simulink model "AcO_Ctrl_Geometric_headless_R2016a"  (R2016a)
settings: Solver=FixedStepDiscrete  StartTime=0.0  StopTime=simulation_duration  FixedStep=Ts  RelTol=1e-3
values from neighbouring files (symbols this model uses):
  M1_BeMo_d = zeros(7,M1_n_mode)    [AcO_Ctrl_headless_cfg.m]    (also in agws_cfg.m = 1e-6*bsxfun(@times,randn(7,M1_n_mode),scale); agws_fastTT_cfg.m = 1e-6*bsxfun(@times,randn(7,M1_n_mode),scale))
  M1_RiBo_d = zeros(7,6)    [AcO_Ctrl_headless_cfg.m]    (also in agws_cfg.m = [M1_Txyz0 M1_Rxyz0]; agws_fastTT_cfg.m = [M1_Txyz0 M1_Rxyz0])
  M2_RiBo_d = zeros(7,6)    [AcO_Ctrl_headless_cfg.m]    (also in agws_cfg.m = [M2_Txyz0 M2_Rxyz0]; agws_fastTT_cfg.m = [M2_Txyz0 M2_Rxyz0])
  Ts = 1/fs    (= 0.002)    [AcO_Ctrl_headless_cfg.m]    (also in agws_fastTT_cfg.m = 0.005)
undefined symbols (not defined in the file or in its folder): Az_C, CG2Hp, CG2Hp_S7, El_C, Fsmm, GIR_C, Hp2CG_f, Hp2CG_f_S7, HPdtf, HpK, KM2, M2_actdyn, M2_CG2Hp, M_LOS, MIMO_C, PTT2act, PTT2act_even, Q, sysd, TT2act, TT2act_even
undefined symbols (not defined in the file): on_axis_src_outputs
libraries: CEO x2
(part 1 of 6)
settings Model: Creator=rconan  LastModifiedBy=rconan
settings DataIOCC: LimitDataPoints=on  SaveFormat=Array
settings OptimizationCC: EfficientMapNaN2IntZero=off
settings HardwareCC: ProdBitPerPointer=32  ProdLargestAtomicFloat=None  ProdIntDivRoundTo=Undefined  ProdEndianess=Unspecified  ProdWordSize=32  ProdHWDeviceType=32-bit Generic  TargetBitPerLong=64  TargetBitPerPointer=64  TargetLongLongMode=on  TargetIntDivRoundTo=Zero  TargetEndianess=LittleEndian  TargetWordSize=64  TargetHWDeviceType=MATLAB Host  ProdEqTarget=off
settings ModelReferenceCC: PropagateSignalLabelsOutOfModel=off
settings CodeAppCC: MaxIdLength=128
settings GRTTargetCC: GeneratePreprocessorConditionals=Use local settings  CombineOutputUpdateFcns=off  GRTInterface=on

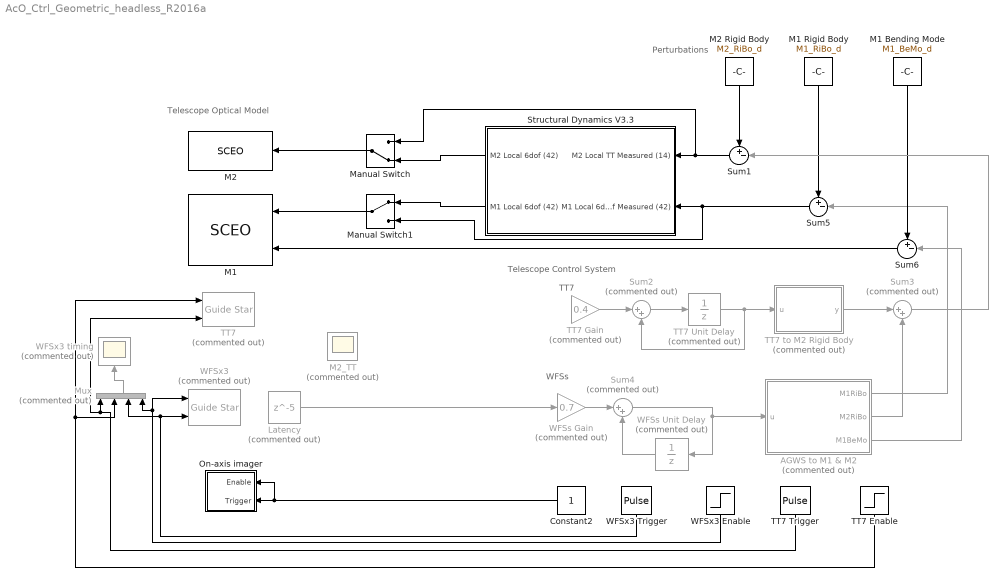
== system AcO_Ctrl_Geometric_headless_R2016a ==
  note: TT7
  note: WFSs
  note: Perturbations
  note: Telescope Control System
  note: Telescope Optical Model
  AGWS to M1 & M2 : MATLAB Function  Commented=on  TreatAsAtomicUnit=on
  Constant2 : Constant  SampleTime=Inf
  Latency : Delay  Commented=on  DelayLength=5
  M1 : M-S-Function  AncestorBlock=CEO/M1 or M2  FunctionName=SCEO  mask(GMTMirror){mirror=M1, TxyzRxyz=on, mode_coefs=on, n_mode=42, sampleTime=[-1,0]}
      mask prompts: TxyzRxyz "Txyz and Rxyz rigid body"; mode_coefs "Mirror mode coefficients"; sampleTime "Sample Time"
      mask help: The GMT M1 or M2 model
      mask init:
      | class_id = 'GMT';
      | msg_box = ceo.dealer(class_id,get_param(gcb,'Name'));
      | set(gcbh,'UserData',msg_box)
      | mask = Simulink.Mask.get(gcb);
      | n_in = 2;
      | msg_box.sampleTime = sampleTime;
      | 
      | gmt_mirror = get_param(gcb,'mirror');
      | 
      | %% START
      | if strcmp(gmt_mirror,'M1')
      |     mirror_args = struct(...
      |         'mirror_modes','bending modes',...
      |         'N_MODE',n_mode);
      |     dims_in = {[7,6],[7,n_mode]};
      | else
      |     mirror_args = struct(...
      |         'mirror_modes','Karhunen-Loeve',...
      |         'N_MODE',n_mode);
      |     dims_in = {[7,6],[7,n_mode]};
      | end
      | start_args = struct('mirror',gmt_mirror,'mirror_args',mirror_args);
      | msg_box.start.args = start_args;
      |          
      | %% UPDATE
      | n_in = 0;
      | inputs_args = struct();
      | update_args = struct('mirror',gmt_mirror,'inputs_args',inputs_args);
      | if TxyzRxyz
      |     n_in = n_in + 1;
      |     dims_in{n_in} = [7,6];
      |     update_args.inputs_args.('TxyzRxyz') = [];
      | end
      | if mode_coefs
      |     n_in = n_in + 1;
      |     dims_in{n_in} = [7,n_mode];
      |     update_args.inputs_args.('mode_coefs') = [];
      | end
      | msg_box.n_in = n_in;
      | msg_box.n_in_ceo = n_in;
      | msg_box.dims_in = dims_in;
      | msg_box.update.args = update_args;
      | 
      | %% OUTPUTS
      | msg_box.n_out = 0;
      | msg_box.dims_out = [];
      mask Help: web(fullfile(fileparts(which('SCEO')),'masks',[get_param(gcb,'MaskType'),'.html']))
      mask TypeOptions mirror: M1 | M2
      mask DialogControl DescGroupVar Prompt: GMT M1 or M2 segmented mirror
      mask DialogControl DescTextVar Prompt: Select to command either M1 or M2 degrees of freedom
      mask DialogControl mirror_commnand Prompt: Mirror commands
      mask Display: fprintf('GMT\nMirror')
  M1 Bending Mode : Constant  Value=M1_BeMo_d
  M1 Rigid Body : Constant  Value=M1_RiBo_d
  M2 : M-S-Function  AncestorBlock=CEO/M1 or M2  FunctionName=SCEO  mask(GMTMirror){mirror=M2, TxyzRxyz=on, mode_coefs=off, n_mode=66, sampleTime=[-1,0]}
      mask prompts: TxyzRxyz "Txyz and Rxyz rigid body"; mode_coefs "Mirror mode coefficients"; sampleTime "Sample Time"
      mask help: The GMT M1 or M2 model
      mask init: same as AcO_Ctrl_Geometric_headless_R2016a/M1
      mask Help: web(fullfile(fileparts(which('SCEO')),'masks',[get_param(gcb,'MaskType'),'.html']))
      mask TypeOptions mirror: M1 | M2
      mask DialogControl DescGroupVar Prompt: GMT M1 or M2 segmented mirror
      mask DialogControl DescTextVar Prompt: Select to command either M1 or M2 degrees of freedom
      mask DialogControl mirror_commnand Prompt: Mirror commands
      mask Display: fprintf('GMT\nMirror')
  M2 Rigid Body : Constant  Value=M2_RiBo_d
  M2_TT : Scope  Commented=on
  Manual Switch : ManualSwitch  CurrentSetting=0
  Manual Switch1 : ManualSwitch
  Mux : Mux  Commented=on
  On-axis imager : Subsystem
  Structural Dynamics V3.3 : Subsystem  Variant=on
  Sum1 : Sum  Inputs=+-|
  Sum2 : Sum  Commented=on  Inputs=|++
  Sum3 : Sum  Commented=on  Inputs=|++
  Sum4 : Sum  Commented=on  Inputs=|++
  Sum5 : Sum  Inputs=+-|
  Sum6 : Sum  Inputs=+-|
  TT7 : CEO/Guide Star  Commented=on  source_prm='JSON/AcO_Ctrl/AcO_TT7_GUIDE_STAR.ubj'  sensor=GeometricTT7  sensor_prm='JSON/AcO_Ctrl/AcO_TT7.ubj'  sensor_calib=tt7_calib  sensor_out={{'M2_TT',14}}  sampleTime=[Ts,0]
  TT7 Trigger : DiscretePulseGenerator  Period=3  PhaseDelay=1/Ts + 3  SampleTime=Ts
  TT7 Enable : Step  SampleTime=Ts
  TT7 Gain : Gain  Commented=on  Gain=0.4
  TT7 Unit Delay : UnitDelay  Commented=on  SampleTime=-1
  TT7 to M2 Rigid Body : MATLAB Function  Commented=on  TreatAsAtomicUnit=on
  WFSs Unit Delay : UnitDelay  Commented=on  SampleTime=-1
  WFSs Gain : Gain  Commented=on  Gain=0.7
  WFSx3 : CEO/Guide Star  Commented=on  source_prm='JSON/AcO_Ctrl/AcO_WFS_GUIDE_STARS.ubj'  sensor=GeometricShackHartmann  sensor_prm='JSON/AcO_Ctrl/AcO_WFS.ubj'  sensor_calib=gs_calib  sensor_out={{'AGWS_D',gs_calib_size}}  sampleTime=[Ts,0]
  WFSx3 Enable : Step  Time=1.5  SampleTime=Ts
  WFSx3 Trigger : DiscretePulseGenerator  Period=0.5/Ts  PhaseDelay=2/Ts  SampleTime=Ts
  WFSx3 timing : Scope  Commented=on
  wires:
  TT7 Unit Delay/1 -> Sum2/2, TT7 to M2 Rigid Body/1(u)
  Sum2/1 -> TT7 Unit Delay/1
  TT7 Gain/1 -> Sum2/1
  Constant2/1 -> On-axis imager/1(Enable), On-axis imager/2(Trigger)
  Mux/1 -> WFSx3 timing/1
  TT7 Trigger/1 -> TT7/2, Mux/1
  TT7 to M2 Rigid Body/1(y) -> Sum3/1
  AGWS to M1 & M2/2(M2RiBo) -> Sum3/2
  Sum4/1 -> WFSs Unit Delay/1, AGWS to M1 & M2/1(u)
  ? -> Latency/1  "AGWS_D"
  WFSs Gain/1 -> Sum4/1
  AGWS to M1 & M2/1(M1RiBo) -> Sum5/2
  M1 Rigid Body/1 -> Sum5/1
  WFSx3 Enable/1 -> Mux/4, WFSx3/1
  AGWS to M1 & M2/3(M1BeMo) -> Sum6/2
  M1 Bending Mode/1 -> Sum6/1
  WFSx3 Trigger/1 -> Mux/3, WFSx3/2
  ? -> TT7 Gain/1, M2_TT/1  "M2_TT"
  Latency/1 -> WFSs Gain/1
  WFSs Unit Delay/1 -> Sum4/2
  Sum5/1 -> Manual Switch1/2, Structural Dynamics V3.3/2(M1 Local 6dof Measured (42))
  Manual Switch/1 -> M2/1
  Manual Switch1/1 -> M1/1
  Sum1/1 -> Manual Switch/1, Structural Dynamics V3.3/1(M2 Local TT Measured (14))
  M2 Rigid Body/1 -> Sum1/1
  TT7 Enable/1 -> Mux/2, TT7/1
  Structural Dynamics V3.3/1(M2 Local 6dof (42)) -> Manual Switch/2
  Structural Dynamics V3.3/2(M1 Local 6dof (42)) -> Manual Switch1/1
  Sum3/1 -> Sum1/2
  Sum6/1 -> M1/2

== system AcO_Ctrl_Geometric_headless_R2016a/On-axis imager ==
  Enable : Inport  SampleTime=Ts
  Trigger : Inport  Port=2  SampleTime=Ts
  Bus Creator : BusCreator  Inputs=5
  Science Star : M-S-Function  AncestorBlock=CEO/Guide Star  FunctionName=SCEO  mask(OpticalPath){source_prm='JSON/AcO_Ctrl/AcO_ON_AXIS_SRC.ubj', sensor=Imaging, sensor_prm='JSON/AcO_Ctrl/AcO_ON_AXIS_IMGR.ubj', sensor_calib=struct('calibrations',[],'filename',[],'pseudo_inverse',[]), sensor_out=on_axis_src_outputs, sampleTime=[Ts,0]}
      mask prompts: source_prm "Parameters"; sensor "Type"; sensor_prm "Parameters"; sensor_calib "Calibration"; sensor_out "Outputs"; sampleTime "Sample Time"
      mask help: Generate a Guide Star and an optional optical sensor
      mask init:
      | class_id = 'OP';
      | msg_box = ceo.dealer(class_id,get_param(gcb,'Name'));
      | set(gcbh,'UserData',msg_box)
      | mask = Simulink.Mask.get(gcb);
      | n_in = 2;
      | dims_in = [];
      | msg_box.n_in = n_in;
      | msg_box.n_in_ceo = 0;
      | msg_box.dims_in = {1,1};
      | n_out = 0;
      | dims_out = {};
      | msg_box.sampleTime = sampleTime;
      | %% START
      | % Source
      | source_args = ceo.liftprm(source_prm);
      | % Sensor
      | prm = mask.getParameter('sensor');
      | sensor_class = prm.TypeOptions{sensor};
      | sensor_args = ceo.liftprm(sensor_prm);
      | miscellaneous_args = [];
      | calib_src_args = [];
      | start_args = struct('source_args',source_args,...
      |               'sensor_class',sensor_class,...
      |               'sensor_args',sensor_args,...
      |               'calibration_source_args',calib_src_args,...
      |               'miscellaneous_args',miscellaneous_args);
      | msg_box.start.args = start_args;
      | %% UPDATE
      | update_args = struct('inputs',[]);
      | msg_box.update.args = update_args;
      | %% OUTPUTS
      | if isempty(sensor_out)
      |     outputs_args = struct('outputs',{[]});
      | else
      |     outputs_args = struct('outputs',{cellfun(@(x) x(1) , sensor_out)} );
      |     dims_out = cellfun(@(x) x(2) , sensor_out );
      |     n_out = numel(dims_out);
      | end
      | msg_box.n_out = n_out;
      | msg_box.dims_out = dims_out;
      | msg_box.outputs.args = outputs_args;
      | %% INITIALIZECONDITIONS
      | init_args = ceo.liftprm(sensor_calib);
      | msg_box.init.args = init_args;
      | 
      | dump(msg_box)
      mask Help: web(fullfile(fileparts(which('SCEO')),'masks',[get_param(gcb,'MaskType'),'.html']))
      mask TypeOptions sensor: None | Imaging | ShackHartmann | GeometricShackHartmann | GeometricTT7
      mask DialogControl DescGroupVar Prompt: Optical Path
      mask DialogControl DescTextVar Prompt: An optical path through the telescope consists in a star and a sensor. Ray tracing is performed from the star to the exist pupil of the GMT. From the exist pupil, the wavefront of the star is Fourier propagated to the detector plane of the sensor.
      mask DialogControl Container14 Prompt: Source
      mask DialogControl Container18 Prompt: Sensor
      mask Display: fprintf('Optical\nPath')
  To File : ToFile  Filename=metrics_MDL353_CASE2_PATCH4.mat  MatrixName=metrics  SaveFormat=Timeseries
  wires:
  Science Star/3 -> Bus Creator/3  "segment_piston"
  Science Star/5 -> Bus Creator/5  "segment_tiptilt"
  Science Star/2 -> Bus Creator/2  "segment_wfe_rms"
  Science Star/1 -> Bus Creator/1  "wfe_rms"
  Enable/1 -> Science Star/1
  Trigger/1 -> Science Star/2
  Science Star/4 -> Bus Creator/4  "tiptilt"
  Bus Creator/1 -> To File/1

== system AcO_Ctrl_Geometric_headless_R2016a/Structural Dynamics V3.3 ==
  M2 Local TT Measured (14) : Inport
  M1 Local 6dof Measured (42) : Inport  Port=2
  Structural Dynamics V3.1 : Subsystem  VariantControl=STATE_SPACE_MDL==310
  Structural Dynamics V3.3 : Subsystem  VariantControl=STATE_SPACE_MDL==330
  Structural Dynamics V3.3a : Subsystem  VariantControl=STATE_SPACE_MDL==331
  Structural Dynamics V3.5.2 : Subsystem  VariantControl=STATE_SPACE_MDL==352
  Structural Dynamics V3.5.3 : Subsystem  VariantControl=STATE_SPACE_MDL==353
  M2 Local 6dof (42) : Outport
  M1 Local 6dof (42) : Outport  Port=2

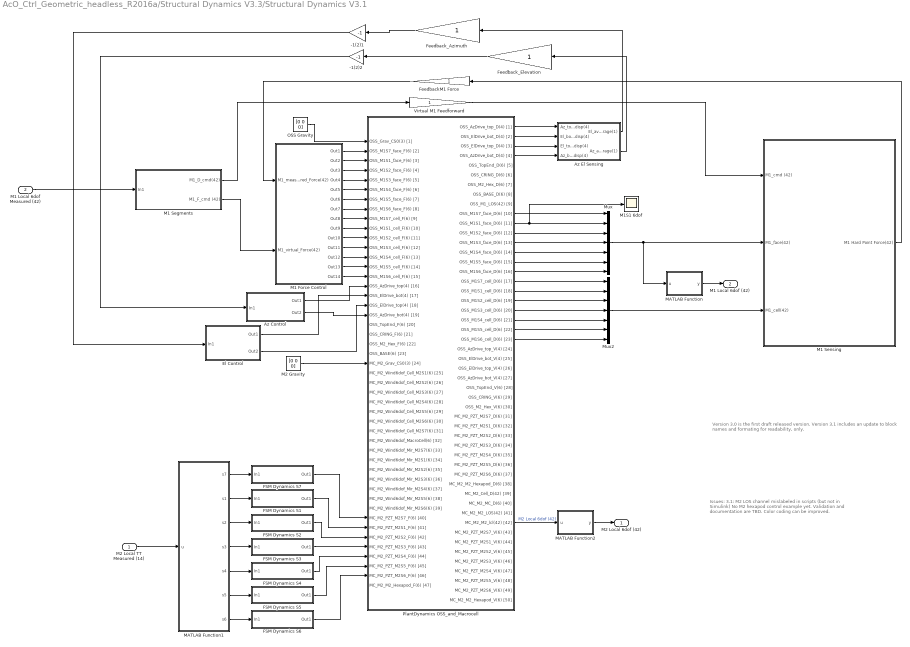
== system AcO_Ctrl_Geometric_headless_R2016a/Structural Dynamics V3.3/Structural Dynamics V3.1 ==
  note: Version 3.0 is  the first draft released version.
      | Version 3.1 includes an update to block names and formating for readability, only.
  note: Issues:
      | 3.1:
      | M2 LOS channel mislabeled in scripts (but not in Simulink)
      | No M2 hexapod control example yet.
      | Validation and documentation are TBD.
      | Color coding can be improved.
  M2 Local TT Measured (14) : Inport
  M1 Local 6dof Measured (42) : Inport  Port=2
  -1(2)1 : Gain  Gain=-1
  -1(2)2 : Gain  Gain=-1
  Az Control : Subsystem
  Az El Sensing : Subsystem
  El Control : Subsystem
  FSM Dynamics S1 : Subsystem
  FSM Dynamics S2 : Subsystem
  FSM Dynamics S3 : Subsystem
  FSM Dynamics S4 : Subsystem
  FSM Dynamics S5 : Subsystem
  FSM Dynamics S6 : Subsystem
  FSM Dynamics S7 : Subsystem
  FeedbackM1 Force : Gain
  Feedback_Azimuth : Gain
  Feedback_Elevation : Gain
  M1 Force Control : Subsystem
  M1 Segments : Subsystem
  M1 Sensing : Subsystem
  M1S1 6dof : Scope
  M2 Gravity : Constant  Value=[0 0 0]
  MATLAB Function : MATLAB Function  TreatAsAtomicUnit=on
  MATLAB Function1 : MATLAB Function  TreatAsAtomicUnit=on
  MATLAB Function2 : MATLAB Function  TreatAsAtomicUnit=on
  Mux : Mux  Inputs=6*ones(7,1)
  Mux2 : Mux  Inputs=6*ones(7,1)
  OSS Gravity : Constant  Value=[0 0 0]
  PlantDynamics OSS_and_Macrocell : Subsystem
  Virtual M1 Feedforward : Gain
  M2 Local 6dof (42) : Outport
  M1 Local 6dof (42) : Outport  Port=2
  wires:
  M2 Local TT Measured (14)/1 -> MATLAB Function1/1(u)
  FSM Dynamics S7/1(Out1) -> PlantDynamics OSS_and_Macrocell/40(MC_M2_PZT_M2S7_F(6) [40])
  MATLAB Function2/1(y) -> M2 Local 6dof (42)/1
  MATLAB Function/1(y) -> M1 Local 6dof (42)/1
  M1 Local 6dof Measured (42)/1 -> M1 Segments/1(In1)
  MATLAB Function1/1(s7) -> FSM Dynamics S7/1(In1)
  MATLAB Function1/2(s1) -> FSM Dynamics S1/1(In1)
  MATLAB Function1/3(s2) -> FSM Dynamics S2/1(In1)
  MATLAB Function1/4(s3) -> FSM Dynamics S3/1(In1)
  MATLAB Function1/5(s4) -> FSM Dynamics S4/1(In1)
  MATLAB Function1/6(s5) -> FSM Dynamics S5/1(In1)
  MATLAB Function1/7(s6) -> FSM Dynamics S6/1(In1)
  Virtual M1 Feedforward/1 -> M1 Sensing/1(M1_cmd (42))
  Az El Sensing/2(Az_average(1)) -> Feedback_Elevation/1
  Az El Sensing/1(El_average(1)) -> Feedback_Azimuth/1
  PlantDynamics OSS_and_Macrocell/4(OSS_AzDrive_bot_D(4) [4]) -> Az El Sensing/4(Az_bot_disp(4))
  PlantDynamics OSS_and_Macrocell/3(OSS_ElDrive_top_D(4) [3]) -> Az El Sensing/3(El_top_disp(4))
  PlantDynamics OSS_and_Macrocell/2(OSS_ElDrive_bot_D(4) [2]) -> Az El Sensing/2(El_bottom_disp(4))
  PlantDynamics OSS_and_Macrocell/1(OSS_AzDrive_top_D(4) [1]) -> Az El Sensing/1(Az_top_disp(4))
  M1 Segments/2(M1_F_cmd (42)) -> M1 Force Control/2(M1_virtual_Force(42))
  M1 Segments/1(M1_D_cmd(42)) -> Virtual M1 Feedforward/1
  M1 Force Control/14(Out14) -> PlantDynamics OSS_and_Macrocell/15(OSS_M1S6_cell_F(6) [15])
  M1 Force Control/13(Out13) -> PlantDynamics OSS_and_Macrocell/14(OSS_M1S5_cell_F(6) [14])
  M1 Force Control/12(Out12) -> PlantDynamics OSS_and_Macrocell/13(OSS_M1S4_cell_F(6) [13])
  M1 Force Control/11(Out11) -> PlantDynamics OSS_and_Macrocell/12(OSS_M1S3_cell_F(6) [12])
  M1 Force Control/10(Out10) -> PlantDynamics OSS_and_Macrocell/11(OSS_M1S2_cell_F(6) [11])
  M1 Force Control/9(Out9) -> PlantDynamics OSS_and_Macrocell/10(OSS_M1S1_cell_F(6) [10])
  M1 Force Control/8(Out8) -> PlantDynamics OSS_and_Macrocell/9(OSS_M1S7_cell_F(6) [9])
  M1 Force Control/7(Out7) -> PlantDynamics OSS_and_Macrocell/8(OSS_M1S6_face_F(6) [8])
  M1 Force Control/6(Out6) -> PlantDynamics OSS_and_Macrocell/7(OSS_M1S5_face_F(6) [7])
  M1 Force Control/5(Out5) -> PlantDynamics OSS_and_Macrocell/6(OSS_M1S4_face_F(6) [6])
  M1 Force Control/4(Out4) -> PlantDynamics OSS_and_Macrocell/5(OSS_M1S3_face_F(6) [5])
  M1 Force Control/3(Out3) -> PlantDynamics OSS_and_Macrocell/4(OSS_M1S2_face_F(6) [4])
  M1 Force Control/2(Out2) -> PlantDynamics OSS_and_Macrocell/3(OSS_M1S1_face_F(6) [3])
  M1 Force Control/1(Out1) -> PlantDynamics OSS_and_Macrocell/2(OSS_M1S7_face_F(6) [2])
  FeedbackM1 Force/1 -> M1 Force Control/1(M1_measured_Force(42))
  El Control/2(Out2) -> PlantDynamics OSS_and_Macrocell/18(OSS_ElDrive_top(4) [18])
  El Control/1(Out1) -> PlantDynamics OSS_and_Macrocell/17(OSS_ElDrive_bot(4) [17])
  -1(2)1/1 -> El Control/1(In1)
  Az Control/2(Out2) -> PlantDynamics OSS_and_Macrocell/19(OSS_AzDrive_bot(4) [19])
  Az Control/1(Out1) -> PlantDynamics OSS_and_Macrocell/16(OSS_AzDrive_top(4) [16])
  -1(2)2/1 -> Az Control/1(In1)
  M1 Sensing/1(M1 Hard Point Force(42)) -> FeedbackM1 Force/1
  Mux2/1 -> M1 Sensing/3(M1_cell(42))
  PlantDynamics OSS_and_Macrocell/23(OSS_M1S6_cell_D(6) [23]) -> Mux2/7
  PlantDynamics OSS_and_Macrocell/22(OSS_M1S5_cell_D(6) [22]) -> Mux2/6
  PlantDynamics OSS_and_Macrocell/21(OSS_M1S4_cell_D(6) [21]) -> Mux2/5
  PlantDynamics OSS_and_Macrocell/20(OSS_M1S3_cell_D(6) [20]) -> Mux2/4
  PlantDynamics OSS_and_Macrocell/19(OSS_M1S2_cell_D(6) [19]) -> Mux2/3
  PlantDynamics OSS_and_Macrocell/18(OSS_M1S1_cell_D(6) [18]) -> Mux2/2
  PlantDynamics OSS_and_Macrocell/17(OSS_M1S7_cell_D(6) [17]) -> Mux2/1
  PlantDynamics OSS_and_Macrocell/15(OSS_M1S5_face_D(6) [15]) -> Mux/6
  PlantDynamics OSS_and_Macrocell/12(OSS_M1S2_face_D(6) [12]) -> Mux/3
  PlantDynamics OSS_and_Macrocell/11(OSS_M1S1_face_D(6) [11]) -> Mux/2, M1S1 6dof/1
  PlantDynamics OSS_and_Macrocell/14(OSS_M1S4_face_D(6) [14]) -> Mux/5
  PlantDynamics OSS_and_Macrocell/16(OSS_M1S6_face_D(6) [16]) -> Mux/7
  PlantDynamics OSS_and_Macrocell/13(OSS_M1S3_face_D(6) [13]) -> Mux/4
  PlantDynamics OSS_and_Macrocell/10(OSS_M1S7_face_D(6) [10]) -> Mux/1
  FSM Dynamics S6/1(Out1) -> PlantDynamics OSS_and_Macrocell/46(MC_M2_PZT_M2S6_F(6) [46])
  FSM Dynamics S5/1(Out1) -> PlantDynamics OSS_and_Macrocell/45(MC_M2_PZT_M2S5_F(6) [45])
  FSM Dynamics S4/1(Out1) -> PlantDynamics OSS_and_Macrocell/44(MC_M2_PZT_M2S4_F(6) [44])
  FSM Dynamics S3/1(Out1) -> PlantDynamics OSS_and_Macrocell/43(MC_M2_PZT_M2S3_F(6) [43])
  FSM Dynamics S2/1(Out1) -> PlantDynamics OSS_and_Macrocell/42(MC_M2_PZT_M2S2_F(6) [42])
  FSM Dynamics S1/1(Out1) -> PlantDynamics OSS_and_Macrocell/41(MC_M2_PZT_M2S1_F(6) [41])
  PlantDynamics OSS_and_Macrocell/42(MC_M2_M2_lcl(42) [42]) -> MATLAB Function2/1(u)  "M2 Local 6dof (42)"
  Mux/1 -> M1 Sensing/2(M1_face(42)), MATLAB Function/1(u)
  Feedback_Elevation/1 -> -1(2)2/1
  Feedback_Azimuth/1 -> -1(2)1/1
  M2 Gravity/1 -> PlantDynamics OSS_and_Macrocell/24(MC_M2_Grav_CS0(3) [24])
  OSS Gravity/1 -> PlantDynamics OSS_and_Macrocell/1(OSS_Grav_CS0(3) [1])

== system AcO_Ctrl_Geometric_headless_R2016a/Structural Dynamics V3.3/Structural Dynamics V3.3 ==
  M2 Local TT Measured (14) : Inport
  M1 Local 6dof Measured (42) : Inport  Port=2
  Loads : Subsystem
  MATLAB Function : MATLAB Function  TreatAsAtomicUnit=on
  MATLAB Function1 : MATLAB Function  TreatAsAtomicUnit=on
  MATLAB Function2 : MATLAB Function  TreatAsAtomicUnit=on
  MC_CEO : Constant  Value=[0;0;0;0;0;0]
  Structural Dynamics Plus CL Az El M1 force : Subsystem
  TT2PTT : MATLAB Function  TreatAsAtomicUnit=on
  M2 Local 6dof (42) : Outport
  M1 Local 6dof (42) : Outport  Port=2
  wires:
  MATLAB Function1/1(y) -> M2 Local 6dof (42)/1
  MATLAB Function/1(y) -> M1 Local 6dof (42)/1
  M2 Local TT Measured (14)/1 -> TT2PTT/1(u)
  Structural Dynamics Plus CL Az El M1 force/1(M1_displacement_lcl(42)) -> MATLAB Function/1(u)
  Structural Dynamics Plus CL Az El M1 force/2(M2 Displacement (segment local) (42)) -> MATLAB Function1/1(u)
  M1 Local 6dof Measured (42)/1 -> MATLAB Function2/1(u)
  MC_CEO/1 -> Structural Dynamics Plus CL Az El M1 force/3(M2 Hexapod Reference M2 Local (6))
  TT2PTT/1(y) -> Structural Dynamics Plus CL Az El M1 force/4(Tip Tilt actuator reference (segment Local) (3))
  Loads/1(Out1) -> Structural Dynamics Plus CL Az El M1 force/1(Loads (111))
  MATLAB Function2/1(y) -> Structural Dynamics Plus CL Az El M1 force/2(M1_reference (42))

== system AcO_Ctrl_Geometric_headless_R2016a/Structural Dynamics V3.3/Structural Dynamics V3.3a ==
  M2 Local TT Measured (14) : Inport
  M1 Local 6dof Measured (42) : Inport  Port=2
  Loads : Subsystem
  MATLAB Function : MATLAB Function  TreatAsAtomicUnit=on
  MATLAB Function1 : MATLAB Function  TreatAsAtomicUnit=on
  MATLAB Function2 : MATLAB Function  TreatAsAtomicUnit=on
  MC_CEO : Constant  Value=[0;0;0;0;0;0]
  Structural Dynamics Plus CL Az El M1 force : Subsystem
  TT2PTT : MATLAB Function  TreatAsAtomicUnit=on
  M2 Local 6dof (42) : Outport
  M1 Local 6dof (42) : Outport  Port=2
  wires:
  MATLAB Function1/1(y) -> M2 Local 6dof (42)/1
  MATLAB Function/1(y) -> M1 Local 6dof (42)/1
  M2 Local TT Measured (14)/1 -> TT2PTT/1(u)
  Structural Dynamics Plus CL Az El M1 force/1(M1_displacement_lcl(42)) -> MATLAB Function/1(u)
  Structural Dynamics Plus CL Az El M1 force/2(M2 Displacement (segment local) (42)) -> MATLAB Function1/1(u)
  M1 Local 6dof Measured (42)/1 -> MATLAB Function2/1(u)
  MC_CEO/1 -> Structural Dynamics Plus CL Az El M1 force/3(M2 Hexapod Reference M2 Local (6))
  TT2PTT/1(y) -> Structural Dynamics Plus CL Az El M1 force/4(Tip Tilt actuator reference (segment Local) (3))
  Loads/1(Out1) -> Structural Dynamics Plus CL Az El M1 force/1(Loads (111))
  MATLAB Function2/1(y) -> Structural Dynamics Plus CL Az El M1 force/2(M1_reference (42))

== system AcO_Ctrl_Geometric_headless_R2016a/Structural Dynamics V3.3/Structural Dynamics V3.5.2 ==
  M2 Local TT Measured (14) : Inport
  M1 Local 6dof Measured (42) : Inport  Port=2
  Loads : Constant  Value=zeros(1,141)
  MATLAB Function : MATLAB Function  TreatAsAtomicUnit=on
  MATLAB Function1 : MATLAB Function  TreatAsAtomicUnit=on
  MATLAB Function2 : MATLAB Function  TreatAsAtomicUnit=on
  MC_CEO : Constant  Value=[0;0;0;0;0;0]
  Manual Switch : ManualSwitch
  Structural Dynamics Plus CL Az El M1 force : Subsystem
  TT2PTT : MATLAB Function  TreatAsAtomicUnit=on
  Terminator : Terminator
  Windloads : Subsystem
  M2 Local 6dof (42) : Outport
  M1 Local 6dof (42) : Outport  Port=2
  wires:
  MATLAB Function1/1(y) -> M2 Local 6dof (42)/1
  MATLAB Function/1(y) -> M1 Local 6dof (42)/1
  M2 Local TT Measured (14)/1 -> TT2PTT/1(u)
  Structural Dynamics Plus CL Az El M1 force/1(M1_displacement_lcl(42)) -> MATLAB Function/1(u)
  Structural Dynamics Plus CL Az El M1 force/2(M2 Displacement (segment local) (42)) -> MATLAB Function1/1(u)
  M1 Local 6dof Measured (42)/1 -> MATLAB Function2/1(u)
  MC_CEO/1 -> Structural Dynamics Plus CL Az El M1 force/3(M2 Hexapod Reference M2 Local (6))
  TT2PTT/1(y) -> Structural Dynamics Plus CL Az El M1 force/4(Tip Tilt actuator reference (segment Local) (3))
  MATLAB Function2/1(y) -> Structural Dynamics Plus CL Az El M1 force/2(M1_reference (42))
  Manual Switch/1 -> Structural Dynamics Plus CL Az El M1 force/1(Loads (141))
  Windloads/1(LoadInputs) -> Manual Switch/1
  Structural Dynamics Plus CL Az El M1 force/3(LOS output (21)) -> Terminator/1
  Loads/1 -> Manual Switch/2

== system AcO_Ctrl_Geometric_headless_R2016a/Structural Dynamics V3.3/Structural Dynamics V3.5.3 ==
  M2 Local TT Measured (14) : Inport
  M1 Local 6dof Measured (42) : Inport  Port=2
  Loads : Constant  Value=zeros(1,141)
  MATLAB Function : MATLAB Function  TreatAsAtomicUnit=on
  MATLAB Function1 : MATLAB Function  TreatAsAtomicUnit=on
  MATLAB Function2 : MATLAB Function  TreatAsAtomicUnit=on
  MC_CEO : Constant  Value=[0;0;0;0;0;0]
  Manual Switch : ManualSwitch
  Structural Dynamics Plus CL Az El M1 force : Subsystem
  TT2PTT : MATLAB Function  TreatAsAtomicUnit=on
  Terminator : Terminator
  Windloads : Subsystem
  M2 Local 6dof (42) : Outport
  M1 Local 6dof (42) : Outport  Port=2
  wires:
  MATLAB Function1/1(y) -> M2 Local 6dof (42)/1
  MATLAB Function/1(y) -> M1 Local 6dof (42)/1
  M2 Local TT Measured (14)/1 -> TT2PTT/1(u)
  Structural Dynamics Plus CL Az El M1 force/1(M1_displacement_lcl(42)) -> MATLAB Function/1(u)
  Structural Dynamics Plus CL Az El M1 force/2(M2 Displacement (segment local) (42)) -> MATLAB Function1/1(u)
  M1 Local 6dof Measured (42)/1 -> MATLAB Function2/1(u)
  MC_CEO/1 -> Structural Dynamics Plus CL Az El M1 force/3(M2 Hexapod Reference M2 Local (6))
  TT2PTT/1(y) -> Structural Dynamics Plus CL Az El M1 force/4(Tip Tilt actuator reference (segment Local) (3))
  MATLAB Function2/1(y) -> Structural Dynamics Plus CL Az El M1 force/2(M1_reference (42))
  Manual Switch/1 -> Structural Dynamics Plus CL Az El M1 force/1(Loads (141))
  Windloads/1(LoadInputs) -> Manual Switch/1
  Structural Dynamics Plus CL Az El M1 force/3(LOS output (21)) -> Terminator/1
  Loads/1 -> Manual Switch/2

== system AcO_Ctrl_Geometric_headless_R2016a/Structural Dynamics V3.3/Structural Dynamics V3.1/Az Control ==
  In1 : Inport
  -1(2) : Gain  Gain=-ones(4,1)  Multiplication=Matrix(K*u)
  Azimuth Controller : DiscreteFilter  Numerator=El_C.num{1}  Denominator=El_C.den{1}  SampleTime=1/Fsmm
  DEMUX1 : Gain  Gain=ones(4,1)  Multiplication=Matrix(K*u)
  Out1 : Outport
  Out2 : Outport  Port=2
  wires:
  -1(2)/1 -> Out2/1
  Azimuth Controller/1 -> DEMUX1/1, -1(2)/1
  DEMUX1/1 -> Out1/1
  In1/1 -> Azimuth Controller/1

== system AcO_Ctrl_Geometric_headless_R2016a/Structural Dynamics V3.3/Structural Dynamics V3.1/Az El Sensing ==
  note: Note: units are m, not radians for these loops!
      | These loops delta the top and bottom displacements in tangential direction, and average the results.
  Az_top_disp(4) : Inport
  El_bottom_disp(4) : Inport  Port=2
  El_top_disp(4) : Inport  Port=3
  Az_bot_disp(4) : Inport  Port=4
  Az : Scope
  El : Scope
  Sum2 : Sum  Inputs=-+|
  Sum3 : Sum  Inputs=-+|
  average : Gain  Gain=ones(1,4)/4  Multiplication=Matrix(K*u)
  average1 : Gain  Gain=ones(1,4)/4  Multiplication=Matrix(K*u)
  El_average(1) : Outport
  Az_average(1) : Outport  Port=2
  wires:
  El_top_disp(4)/1 -> Sum2/2
  El_bottom_disp(4)/1 -> Sum2/1
  Sum2/1 -> average/1
  Sum3/1 -> average1/1
  average1/1 -> Az/1, Az_average(1)/1
  Az_bot_disp(4)/1 -> Sum3/1
  Az_top_disp(4)/1 -> Sum3/2
  average/1 -> El_average(1)/1, El/1

== system AcO_Ctrl_Geometric_headless_R2016a/Structural Dynamics V3.3/Structural Dynamics V3.1/El Control ==
  In1 : Inport
  -1 : Gain  Gain=-ones(4,1)  Multiplication=Matrix(K*u)
  DEMUX : Gain  Gain=ones(4,1)  Multiplication=Matrix(K*u)
  Elevation Controller : DiscreteFilter  Numerator=El_C.num{1}  Denominator=El_C.den{1}  SampleTime=1/Fsmm
  Out1 : Outport
  Out2 : Outport  Port=2
  wires:
  In1/1 -> Elevation Controller/1
  DEMUX/1 -> Out2/1
  -1/1 -> Out1/1
  Elevation Controller/1 -> DEMUX/1, -1/1

== system AcO_Ctrl_Geometric_headless_R2016a/Structural Dynamics V3.3/Structural Dynamics V3.1/FSM Dynamics S1 ==
  In1 : Inport
  M2actuatorDyanmics5 : DiscreteStateSpace  A=M2_actdyn.A  B=M2_actdyn.B  C=M2_actdyn.C  D=M2_actdyn.D  SampleTime=1/Fsmm
  TT_to_act5 : Gain  Gain=TT2act  Multiplication=Matrix(K*u)
  delta1 : Gain  Gain=[eye(3);-eye(3)]  Multiplication=Matrix(K*u)
  Out1 : Outport
  wires:
  delta1/1 -> Out1/1
  TT_to_act5/1 -> M2actuatorDyanmics5/1
  In1/1 -> TT_to_act5/1
  M2actuatorDyanmics5/1 -> delta1/1

== system AcO_Ctrl_Geometric_headless_R2016a/Structural Dynamics V3.3/Structural Dynamics V3.1/FSM Dynamics S2 ==
  In1 : Inport
  M2actuatorDyanmics5 : DiscreteStateSpace  A=M2_actdyn.A  B=M2_actdyn.B  C=M2_actdyn.C  D=M2_actdyn.D  SampleTime=1/Fsmm
  TT_to_act5 : Gain  Gain=TT2act_even  Multiplication=Matrix(K*u)
  delta1 : Gain  Gain=[eye(3);-eye(3)]  Multiplication=Matrix(K*u)
  Out1 : Outport
  wires:
  delta1/1 -> Out1/1
  TT_to_act5/1 -> M2actuatorDyanmics5/1
  In1/1 -> TT_to_act5/1
  M2actuatorDyanmics5/1 -> delta1/1

== system AcO_Ctrl_Geometric_headless_R2016a/Structural Dynamics V3.3/Structural Dynamics V3.1/FSM Dynamics S3 ==
  In1 : Inport
  M2actuatorDyanmics5 : DiscreteStateSpace  A=M2_actdyn.A  B=M2_actdyn.B  C=M2_actdyn.C  D=M2_actdyn.D  SampleTime=1/Fsmm
  TT_to_act5 : Gain  Gain=TT2act  Multiplication=Matrix(K*u)
  delta1 : Gain  Gain=[eye(3);-eye(3)]  Multiplication=Matrix(K*u)
  Out1 : Outport
  wires:
  delta1/1 -> Out1/1
  TT_to_act5/1 -> M2actuatorDyanmics5/1
  In1/1 -> TT_to_act5/1
  M2actuatorDyanmics5/1 -> delta1/1

== system AcO_Ctrl_Geometric_headless_R2016a/Structural Dynamics V3.3/Structural Dynamics V3.1/FSM Dynamics S4 ==
  In1 : Inport
  M2actuatorDyanmics5 : DiscreteStateSpace  A=M2_actdyn.A  B=M2_actdyn.B  C=M2_actdyn.C  D=M2_actdyn.D  SampleTime=1/Fsmm
  TT_to_act5 : Gain  Gain=TT2act_even  Multiplication=Matrix(K*u)
  delta1 : Gain  Gain=[eye(3);-eye(3)]  Multiplication=Matrix(K*u)
  Out1 : Outport
  wires:
  delta1/1 -> Out1/1
  TT_to_act5/1 -> M2actuatorDyanmics5/1
  In1/1 -> TT_to_act5/1
  M2actuatorDyanmics5/1 -> delta1/1

== system AcO_Ctrl_Geometric_headless_R2016a/Structural Dynamics V3.3/Structural Dynamics V3.1/FSM Dynamics S5 ==
  In1 : Inport
  M2actuatorDyanmics5 : DiscreteStateSpace  A=M2_actdyn.A  B=M2_actdyn.B  C=M2_actdyn.C  D=M2_actdyn.D  SampleTime=1/Fsmm
  TT_to_act5 : Gain  Gain=TT2act  Multiplication=Matrix(K*u)
  delta1 : Gain  Gain=[eye(3);-eye(3)]  Multiplication=Matrix(K*u)
  Out1 : Outport
  wires:
  delta1/1 -> Out1/1
  TT_to_act5/1 -> M2actuatorDyanmics5/1
  In1/1 -> TT_to_act5/1
  M2actuatorDyanmics5/1 -> delta1/1

== system AcO_Ctrl_Geometric_headless_R2016a/Structural Dynamics V3.3/Structural Dynamics V3.1/FSM Dynamics S6 ==
  In1 : Inport
  M2actuatorDyanmics5 : DiscreteStateSpace  A=M2_actdyn.A  B=M2_actdyn.B  C=M2_actdyn.C  D=M2_actdyn.D  SampleTime=1/Fsmm
  TT_to_act5 : Gain  Gain=TT2act_even  Multiplication=Matrix(K*u)
  delta1 : Gain  Gain=[eye(3);-eye(3)]  Multiplication=Matrix(K*u)
  Out1 : Outport
  wires:
  delta1/1 -> Out1/1
  TT_to_act5/1 -> M2actuatorDyanmics5/1
  In1/1 -> TT_to_act5/1
  M2actuatorDyanmics5/1 -> delta1/1

== system AcO_Ctrl_Geometric_headless_R2016a/Structural Dynamics V3.3/Structural Dynamics V3.1/FSM Dynamics S7 ==
  In1 : Inport
  M2actuatorDyanmics5 : DiscreteStateSpace  A=M2_actdyn.A  B=M2_actdyn.B  C=M2_actdyn.C  D=M2_actdyn.D  SampleTime=1/Fsmm
  TT_to_act5 : Gain  Gain=TT2act  Multiplication=Matrix(K*u)
  delta1 : Gain  Gain=[eye(3);-eye(3)]  Multiplication=Matrix(K*u)
  Out1 : Outport
  wires:
  delta1/1 -> Out1/1
  TT_to_act5/1 -> M2actuatorDyanmics5/1
  In1/1 -> TT_to_act5/1
  M2actuatorDyanmics5/1 -> delta1/1

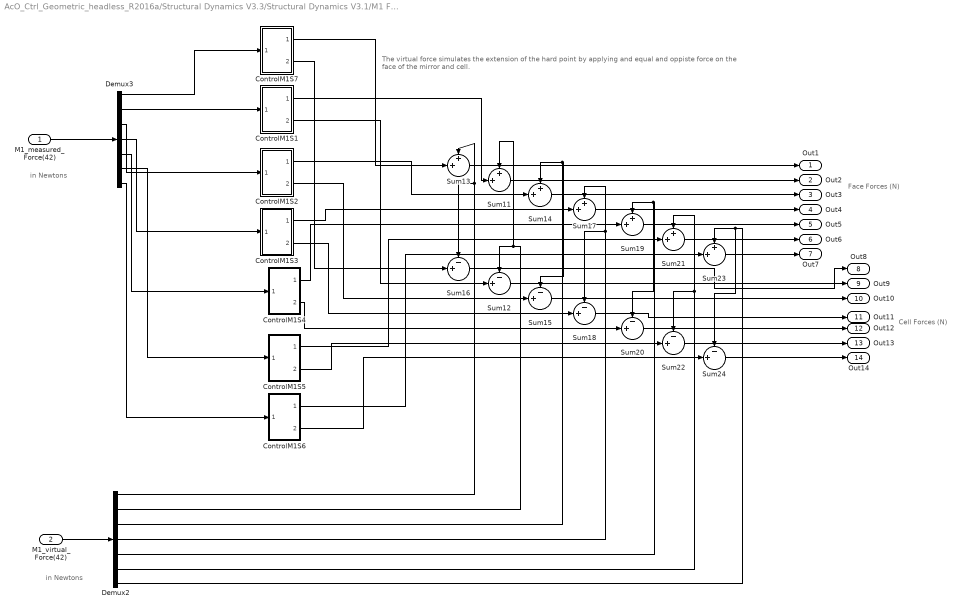
== system AcO_Ctrl_Geometric_headless_R2016a/Structural Dynamics V3.3/Structural Dynamics V3.1/M1 Force Control ==
  note: Face Forces (N)
  note: Cell Forces (N)
  note: The virtual force simulates the extension of the hard point by applying and equal and oppiste force on the face of the mirror and cell.
  note: in Newtons
  note: in Newtons
  M1_measured_Force(42) : Inport
  M1_virtual_Force(42) : Inport  Port=2
  ControlM1S1 : Subsystem
  ControlM1S2 : Subsystem
  ControlM1S3 : Subsystem
  ControlM1S4 : Subsystem
  ControlM1S5 : Subsystem
  ControlM1S6 : Subsystem
  ControlM1S7 : Subsystem
  Demux2 : Demux  Outputs=6*ones(7,1)
  Demux3 : Demux  Outputs=6*ones(7,1)
  Sum{11,13..14,17,19,21,23} (7 alike) : Sum  Inputs=++|
  Sum{12,15..16,18,20,22,24} (7 alike) : Sum  Inputs=-+|
  Out1 : Outport
  Out2 : Outport  Port=2
  Out3 : Outport  Port=3
  Out4 : Outport  Port=4
  Out5 : Outport  Port=5
  Out6 : Outport  Port=6
  Out7 : Outport  Port=7
  Out8 : Outport  Port=8
  Out9 : Outport  Port=9
  Out10 : Outport  Port=10
  Out11 : Outport  Port=11
  Out12 : Outport  Port=12
  Out13 : Outport  Port=13
  Out14 : Outport  Port=14
  wires:
  M1_virtual_Force(42)/1 -> Demux2/1
  ControlM1S7/1(Out1) -> Sum13/2
  Demux2/2 -> Sum11/1, Sum12/1
  ControlM1S6/2(Out2) -> Sum24/2
  Demux2/7 -> Sum24/1, Sum23/1
  ControlM1S5/2(Out2) -> Sum22/2
  Demux2/5 -> Sum20/1, Sum19/1
  Demux2/1 -> Sum16/1, Sum13/1
  Demux3/6 -> ControlM1S5/1(In1)
  Demux3/7 -> ControlM1S6/1(In1)
  ControlM1S7/2(Out2) -> Sum16/2
  Demux2/3 -> Sum15/1, Sum14/1
  ControlM1S4/2(Out2) -> Sum20/2
  Demux2/4 -> Sum18/1, Sum17/1
  Demux2/6 -> Sum22/1, Sum21/1
  Demux3/2 -> ControlM1S1/1(In1)
  Demux3/1 -> ControlM1S7/1(In1)
  Demux3/4 -> ControlM1S3/1(In1)
  Demux3/3 -> ControlM1S2/1(In1)
  Demux3/5 -> ControlM1S4/1(In1)
  ControlM1S3/1(Out1) -> Sum17/2
  ControlM1S2/1(Out1) -> Sum14/2
  ControlM1S1/2(Out2) -> Sum12/2
  ControlM1S5/1(Out1) -> Sum21/2
  ControlM1S2/2(Out2) -> Sum15/2
  ControlM1S3/2(Out2) -> Sum18/2
  ControlM1S6/1(Out1) -> Sum23/2
  ControlM1S1/1(Out1) -> Sum11/2
  ControlM1S4/1(Out1) -> Sum19/2
  Sum14/1 -> Out3/1
  Sum11/1 -> Out2/1
  Sum19/1 -> Out5/1
  Sum17/1 -> Out4/1
  Sum18/1 -> Out11/1
  Sum15/1 -> Out10/1
  Sum12/1 -> Out9/1
  Sum20/1 -> Out12/1
  Sum24/1 -> Out14/1
  Sum23/1 -> Out7/1
  Sum21/1 -> Out6/1
  Sum22/1 -> Out13/1
  Sum16/1 -> Out8/1
  Sum13/1 -> Out1/1
  M1_measured_Force(42)/1 -> Demux3/1

== system AcO_Ctrl_Geometric_headless_R2016a/Structural Dynamics V3.3/Structural Dynamics V3.1/M1 Segments ==
  In1 : Inport
  KHp{1..7} (7 alike) : Gain  Gain=HpK  Multiplication=Matrix(K*u)
  MATLAB Function : MATLAB Function  TreatAsAtomicUnit=on
  Mux1 : Mux  Inputs=6*ones(7,1)
  Mux3 : Mux  Inputs=6*ones(7,1)
  M1_D_cmd(42) : Outport
  M1_F_cmd (42) : Outport  Port=2
  wires:
  Mux3/1 -> M1_D_cmd(42)/1
  Mux1/1 -> M1_F_cmd (42)/1
  KHp3/1 -> Mux1/3
  MATLAB Function/2(s1) -> KHp1/1, Mux3/2
  KHp1/1 -> Mux1/2
  KHp5/1 -> Mux1/5
  KHp4/1 -> Mux1/4
  KHp6/1 -> Mux1/6
  MATLAB Function/1(s7) -> KHp2/1, Mux3/1
  KHp2/1 -> Mux1/1
  In1/1 -> MATLAB Function/1(u)
  MATLAB Function/3(s2) -> KHp3/1, Mux3/3
  MATLAB Function/6(s5) -> KHp6/1, Mux3/6
  MATLAB Function/4(s3) -> KHp4/1, Mux3/4
  KHp7/1 -> Mux1/7
  MATLAB Function/5(s4) -> KHp5/1, Mux3/5
  MATLAB Function/7(s6) -> KHp7/1, Mux3/7

== system AcO_Ctrl_Geometric_headless_R2016a/Structural Dynamics V3.3/Structural Dynamics V3.1/M1 Sensing ==
  M1_cmd (42) : Inport
  M1_face(42) : Inport  Port=2
  M1_cell(42) : Inport  Port=3
  Demux1 : Demux  Outputs=6*ones(7,1)
  Demux2 : Demux  Outputs=6*ones(7,1)
  Demux9 : Demux  Outputs=6*ones(7,1)
  Mux3 : Mux  Inputs=6*ones(7,1)
  senseM1S1 : Subsystem
  senseM1S2 : Subsystem
  senseM1S3 : Subsystem
  senseM1S4 : Subsystem
  senseM1S5 : Subsystem
  senseM1S6 : Subsystem
  senseM1S7 : Subsystem
  M1 Hard Point Force(42) : Outport
  wires:
  M1_face(42)/1 -> Demux1/1
  Demux9/7 -> senseM1S6/1(6dof_D_cmd)
  Demux9/5 -> senseM1S4/1(6dof_D_cmd)
  Demux9/1 -> senseM1S7/1(6dof_D_cmd)
  Demux9/6 -> senseM1S5/1(6dof_D_cmd)
  Demux9/4 -> senseM1S3/1(6dof_D_cmd)
  M1_cmd (42)/1 -> Demux9/1
  Demux9/3 -> senseM1S2/1(6dof_D_cmd)
  Demux1/3 -> senseM1S2/2(6dof_D_face)
  Demux1/2 -> senseM1S1/2(6dof_D_face)
  Demux9/2 -> senseM1S1/1(6dof_D_cmd)
  Mux3/1 -> M1 Hard Point Force(42)/1
  senseM1S6/1(HardPointForce) -> Mux3/7
  Demux1/6 -> senseM1S5/2(6dof_D_face)
  Demux1/7 -> senseM1S6/2(6dof_D_face)
  Demux2/1 -> senseM1S7/3(6dof_D_cell)
  M1_cell(42)/1 -> Demux2/1
  senseM1S2/1(HardPointForce) -> Mux3/3
  senseM1S3/1(HardPointForce) -> Mux3/4
  senseM1S4/1(HardPointForce) -> Mux3/5
  Demux1/1 -> senseM1S7/2(6dof_D_face)
  Demux2/6 -> senseM1S5/3(6dof_D_cell)
  Demux2/7 -> senseM1S6/3(6dof_D_cell)
  senseM1S7/1(HardPointForce) -> Mux3/1
  senseM1S5/1(HardPointForce) -> Mux3/6
  Demux1/5 -> senseM1S4/2(6dof_D_face)
  Demux2/4 -> senseM1S3/3(6dof_D_cell)
  Demux2/3 -> senseM1S2/3(6dof_D_cell)
  Demux2/2 -> senseM1S1/3(6dof_D_cell)
  senseM1S1/1(HardPointForce) -> Mux3/2
  Demux1/4 -> senseM1S3/2(6dof_D_face)
  Demux2/5 -> senseM1S4/3(6dof_D_cell)

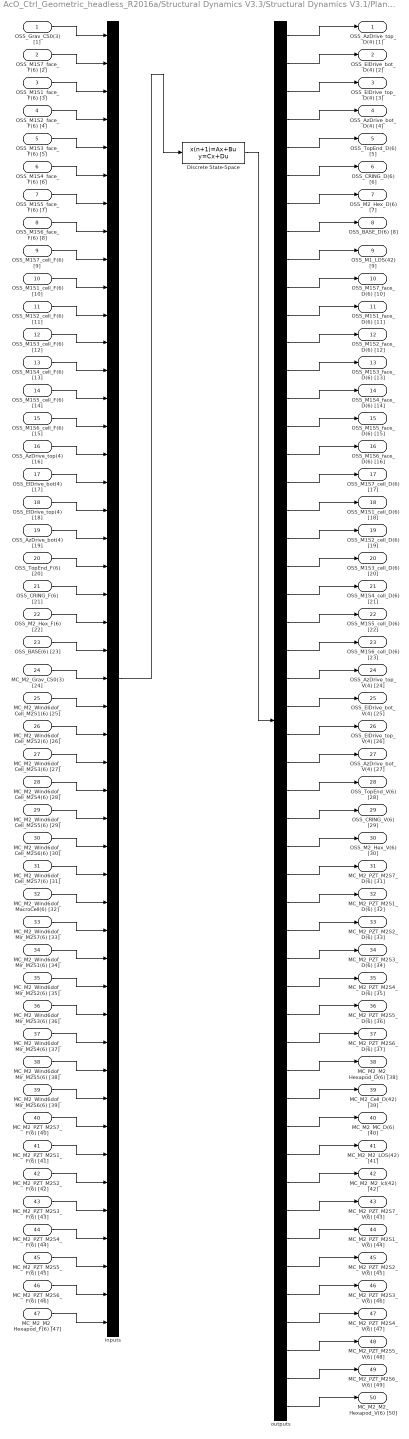
== system AcO_Ctrl_Geometric_headless_R2016a/Structural Dynamics V3.3/Structural Dynamics V3.1/PlantDynamics OSS_and_Macrocell ==
  OSS_Grav_CS0(3) [1] : Inport  PortDimensions=3
  OSS_M1S7_face_F(6) [2] : Inport  Port=2  PortDimensions=6
  OSS_M1S1_face_F(6) [3] : Inport  Port=3  PortDimensions=6
  OSS_M1S2_face_F(6) [4] : Inport  Port=4  PortDimensions=6
  OSS_M1S3_face_F(6) [5] : Inport  Port=5  PortDimensions=6
  OSS_M1S4_face_F(6) [6] : Inport  Port=6  PortDimensions=6
  OSS_M1S5_face_F(6) [7] : Inport  Port=7  PortDimensions=6
  OSS_M1S6_face_F(6) [8] : Inport  Port=8  PortDimensions=6
  OSS_M1S7_cell_F(6) [9] : Inport  Port=9  PortDimensions=6
  OSS_M1S1_cell_F(6) [10] : Inport  Port=10  PortDimensions=6
  OSS_M1S2_cell_F(6) [11] : Inport  Port=11  PortDimensions=6
  OSS_M1S3_cell_F(6) [12] : Inport  Port=12  PortDimensions=6
  OSS_M1S4_cell_F(6) [13] : Inport  Port=13  PortDimensions=6
  OSS_M1S5_cell_F(6) [14] : Inport  Port=14  PortDimensions=6
  OSS_M1S6_cell_F(6) [15] : Inport  Port=15  PortDimensions=6
  OSS_AzDrive_top(4) [16] : Inport  Port=16  PortDimensions=4
  OSS_ElDrive_bot(4) [17] : Inport  Port=17  PortDimensions=4
  OSS_ElDrive_top(4) [18] : Inport  Port=18  PortDimensions=4
  OSS_AzDrive_bot(4) [19] : Inport  Port=19  PortDimensions=4
  OSS_TopEnd_F(6) [20] : Inport  Port=20  PortDimensions=6
  OSS_CRING_F(6) [21] : Inport  Port=21  PortDimensions=6
  OSS_M2_Hex_F(6) [22] : Inport  Port=22  PortDimensions=6
  OSS_BASE(6) [23] : Inport  Port=23  PortDimensions=6
  MC_M2_Grav_CS0(3) [24] : Inport  Port=24  PortDimensions=3
  MC_M2_Wind6dof_Cell_M2S1(6) [25] : Inport  Port=25  PortDimensions=6
  MC_M2_Wind6dof_Cell_M2S2(6) [26] : Inport  Port=26  PortDimensions=6
  MC_M2_Wind6dof_Cell_M2S3(6) [27] : Inport  Port=27  PortDimensions=6
  MC_M2_Wind6dof_Cell_M2S4(6) [28] : Inport  Port=28  PortDimensions=6
  MC_M2_Wind6dof_Cell_M2S5(6) [29] : Inport  Port=29  PortDimensions=6
  MC_M2_Wind6dof_Cell_M2S6(6) [30] : Inport  Port=30  PortDimensions=6
  MC_M2_Wind6dof_Cell_M2S7(6) [31] : Inport  Port=31  PortDimensions=6
  MC_M2_Wind6dof_MacroCell(6) [32] : Inport  Port=32  PortDimensions=6
  MC_M2_Wind6dof_Mir_M2S7(6) [33] : Inport  Port=33  PortDimensions=6
  MC_M2_Wind6dof_Mir_M2S1(6) [34] : Inport  Port=34  PortDimensions=6
  MC_M2_Wind6dof_Mir_M2S2(6) [35] : Inport  Port=35  PortDimensions=6
  MC_M2_Wind6dof_Mir_M2S3(6) [36] : Inport  Port=36  PortDimensions=6
  MC_M2_Wind6dof_Mir_M2S4(6) [37] : Inport  Port=37  PortDimensions=6
  MC_M2_Wind6dof_Mir_M2S5(6) [38] : Inport  Port=38  PortDimensions=6
  MC_M2_Wind6dof_Mir_M2S6(6) [39] : Inport  Port=39  PortDimensions=6
  MC_M2_PZT_M2S7_F(6) [40] : Inport  Port=40  PortDimensions=6
  MC_M2_PZT_M2S1_F(6) [41] : Inport  Port=41  PortDimensions=6
  MC_M2_PZT_M2S2_F(6) [42] : Inport  Port=42  PortDimensions=6
  MC_M2_PZT_M2S3_F(6) [43] : Inport  Port=43  PortDimensions=6
  MC_M2_PZT_M2S4_F(6) [44] : Inport  Port=44  PortDimensions=6
  MC_M2_PZT_M2S5_F(6) [45] : Inport  Port=45  PortDimensions=6
  MC_M2_PZT_M2S6_F(6) [46] : Inport  Port=46  PortDimensions=6
  MC_M2_M2_Hexapod_F(6) [47] : Inport  Port=47  PortDimensions=6
  Discrete State-Space : DiscreteStateSpace  A=sysd.sys.A  B=sysd.sys.B  C=sysd.sys.C  D=sysd.sys.D  SampleTime=sysd.sys.Ts
  inputs : Mux  Inputs=[3,6,6,6,6,6,6,6,6,6,6,6,6,6,6,4,4,4,4,6,6,6,6,3,6,6,6,6,6,6,6,6,6,6,6,6,6,6,6,6,6,6,6,6,6,6,6]
  outputs : Demux  Outputs=[4,4,4,4,6,6,6,6,42,6,6,6,6,6,6,6,6,6,6,6,6,6,6,4,4,4,4,6,6,6,6,6,6,6,6,6,6,6,42,6,42,42,6,6,6,6,6,6,6,6]
  OSS_AzDrive_top_D(4) [1] : Outport  PortDimensions=4
  OSS_ElDrive_bot_D(4) [2] : Outport  Port=2  PortDimensions=4
  OSS_ElDrive_top_D(4) [3] : Outport  Port=3  PortDimensions=4
  OSS_AzDrive_bot_D(4) [4] : Outport  Port=4  PortDimensions=4
  OSS_TopEnd_D(6) [5] : Outport  Port=5  PortDimensions=6
  OSS_CRING_D(6) [6] : Outport  Port=6  PortDimensions=6
  OSS_M2_Hex_D(6) [7] : Outport  Port=7  PortDimensions=6
  OSS_BASE_D(6) [8] : Outport  Port=8  PortDimensions=6
  OSS_M1_LOS(42) [9] : Outport  Port=9  PortDimensions=42
  OSS_M1S7_face_D(6) [10] : Outport  Port=10  PortDimensions=6
  OSS_M1S1_face_D(6) [11] : Outport  Port=11  PortDimensions=6
  OSS_M1S2_face_D(6) [12] : Outport  Port=12  PortDimensions=6
  OSS_M1S3_face_D(6) [13] : Outport  Port=13  PortDimensions=6
  OSS_M1S4_face_D(6) [14] : Outport  Port=14  PortDimensions=6
  OSS_M1S5_face_D(6) [15] : Outport  Port=15  PortDimensions=6
  OSS_M1S6_face_D(6) [16] : Outport  Port=16  PortDimensions=6
  OSS_M1S7_cell_D(6) [17] : Outport  Port=17  PortDimensions=6
  OSS_M1S1_cell_D(6) [18] : Outport  Port=18  PortDimensions=6
  OSS_M1S2_cell_D(6) [19] : Outport  Port=19  PortDimensions=6
  OSS_M1S3_cell_D(6) [20] : Outport  Port=20  PortDimensions=6
  OSS_M1S4_cell_D(6) [21] : Outport  Port=21  PortDimensions=6
  OSS_M1S5_cell_D(6) [22] : Outport  Port=22  PortDimensions=6
  OSS_M1S6_cell_D(6) [23] : Outport  Port=23  PortDimensions=6
  OSS_AzDrive_top_V(4) [24] : Outport  Port=24  PortDimensions=4
  OSS_ElDrive_bot_V(4) [25] : Outport  Port=25  PortDimensions=4
  OSS_ElDrive_top_V(4) [26] : Outport  Port=26  PortDimensions=4
  OSS_AzDrive_bot_V(4) [27] : Outport  Port=27  PortDimensions=4
  OSS_TopEnd_V(6) [28] : Outport  Port=28  PortDimensions=6
  OSS_CRING_V(6) [29] : Outport  Port=29  PortDimensions=6
  OSS_M2_Hex_V(6) [30] : Outport  Port=30  PortDimensions=6
  MC_M2_PZT_M2S7_D(6) [31] : Outport  Port=31  PortDimensions=6
  MC_M2_PZT_M2S1_D(6) [32] : Outport  Port=32  PortDimensions=6
  MC_M2_PZT_M2S2_D(6) [33] : Outport  Port=33  PortDimensions=6
  MC_M2_PZT_M2S3_D(6) [34] : Outport  Port=34  PortDimensions=6
  MC_M2_PZT_M2S4_D(6) [35] : Outport  Port=35  PortDimensions=6
  MC_M2_PZT_M2S5_D(6) [36] : Outport  Port=36  PortDimensions=6
  MC_M2_PZT_M2S6_D(6) [37] : Outport  Port=37  PortDimensions=6
  MC_M2_M2_Hexapod_D(6) [38] : Outport  Port=38  PortDimensions=6
  MC_M2_Cell_D(42) [39] : Outport  Port=39  PortDimensions=42
  MC_M2_MC_D(6) [40] : Outport  Port=40  PortDimensions=6
  MC_M2_M2_LOS(42) [41] : Outport  Port=41  PortDimensions=42
  MC_M2_M2_lcl(42) [42] : Outport  Port=42  PortDimensions=42
  MC_M2_PZT_M2S7_V(6) [43] : Outport  Port=43  PortDimensions=6
  MC_M2_PZT_M2S1_V(6) [44] : Outport  Port=44  PortDimensions=6
  MC_M2_PZT_M2S2_V(6) [45] : Outport  Port=45  PortDimensions=6
  MC_M2_PZT_M2S3_V(6) [46] : Outport  Port=46  PortDimensions=6
  MC_M2_PZT_M2S4_V(6) [47] : Outport  Port=47  PortDimensions=6
  MC_M2_PZT_M2S5_V(6) [48] : Outport  Port=48  PortDimensions=6
  MC_M2_PZT_M2S6_V(6) [49] : Outport  Port=49  PortDimensions=6
  MC_M2_M2_Hexapod_V(6) [50] : Outport  Port=50  PortDimensions=6
  wires:
  outputs/50 -> MC_M2_M2_Hexapod_V(6) [50]/1
  outputs/49 -> MC_M2_PZT_M2S6_V(6) [49]/1
  outputs/48 -> MC_M2_PZT_M2S5_V(6) [48]/1
  outputs/47 -> MC_M2_PZT_M2S4_V(6) [47]/1
  outputs/46 -> MC_M2_PZT_M2S3_V(6) [46]/1
  outputs/45 -> MC_M2_PZT_M2S2_V(6) [45]/1
  outputs/44 -> MC_M2_PZT_M2S1_V(6) [44]/1
  outputs/43 -> MC_M2_PZT_M2S7_V(6) [43]/1
  outputs/42 -> MC_M2_M2_lcl(42) [42]/1
  outputs/41 -> MC_M2_M2_LOS(42) [41]/1
  outputs/40 -> MC_M2_MC_D(6) [40]/1
  outputs/39 -> MC_M2_Cell_D(42) [39]/1
  outputs/38 -> MC_M2_M2_Hexapod_D(6) [38]/1
  outputs/37 -> MC_M2_PZT_M2S6_D(6) [37]/1
  outputs/36 -> MC_M2_PZT_M2S5_D(6) [36]/1
  outputs/35 -> MC_M2_PZT_M2S4_D(6) [35]/1
  outputs/34 -> MC_M2_PZT_M2S3_D(6) [34]/1
  outputs/33 -> MC_M2_PZT_M2S2_D(6) [33]/1
  outputs/32 -> MC_M2_PZT_M2S1_D(6) [32]/1
  outputs/31 -> MC_M2_PZT_M2S7_D(6) [31]/1
  outputs/30 -> OSS_M2_Hex_V(6) [30]/1
  outputs/29 -> OSS_CRING_V(6) [29]/1
  outputs/28 -> OSS_TopEnd_V(6) [28]/1
  outputs/27 -> OSS_AzDrive_bot_V(4) [27]/1
  outputs/26 -> OSS_ElDrive_top_V(4) [26]/1
  outputs/25 -> OSS_ElDrive_bot_V(4) [25]/1
  outputs/24 -> OSS_AzDrive_top_V(4) [24]/1
  outputs/23 -> OSS_M1S6_cell_D(6) [23]/1
  outputs/22 -> OSS_M1S5_cell_D(6) [22]/1
  outputs/21 -> OSS_M1S4_cell_D(6) [21]/1
  outputs/20 -> OSS_M1S3_cell_D(6) [20]/1
  outputs/19 -> OSS_M1S2_cell_D(6) [19]/1
  outputs/18 -> OSS_M1S1_cell_D(6) [18]/1
  outputs/17 -> OSS_M1S7_cell_D(6) [17]/1
  outputs/16 -> OSS_M1S6_face_D(6) [16]/1
  outputs/15 -> OSS_M1S5_face_D(6) [15]/1
  outputs/14 -> OSS_M1S4_face_D(6) [14]/1
  outputs/13 -> OSS_M1S3_face_D(6) [13]/1
  outputs/12 -> OSS_M1S2_face_D(6) [12]/1
  outputs/11 -> OSS_M1S1_face_D(6) [11]/1
  outputs/10 -> OSS_M1S7_face_D(6) [10]/1
  outputs/9 -> OSS_M1_LOS(42) [9]/1
  outputs/8 -> OSS_BASE_D(6) [8]/1
  outputs/7 -> OSS_M2_Hex_D(6) [7]/1
  outputs/6 -> OSS_CRING_D(6) [6]/1
  outputs/5 -> OSS_TopEnd_D(6) [5]/1
  outputs/4 -> OSS_AzDrive_bot_D(4) [4]/1
  outputs/3 -> OSS_ElDrive_top_D(4) [3]/1
  outputs/2 -> OSS_ElDrive_bot_D(4) [2]/1
  outputs/1 -> OSS_AzDrive_top_D(4) [1]/1
  Discrete State-Space/1 -> outputs/1
  inputs/1 -> Discrete State-Space/1
  MC_M2_M2_Hexapod_F(6) [47]/1 -> inputs/47
  MC_M2_PZT_M2S6_F(6) [46]/1 -> inputs/46
  MC_M2_PZT_M2S5_F(6) [45]/1 -> inputs/45
  MC_M2_PZT_M2S4_F(6) [44]/1 -> inputs/44
  MC_M2_PZT_M2S3_F(6) [43]/1 -> inputs/43
  MC_M2_PZT_M2S2_F(6) [42]/1 -> inputs/42
  MC_M2_PZT_M2S1_F(6) [41]/1 -> inputs/41
  MC_M2_PZT_M2S7_F(6) [40]/1 -> inputs/40
  MC_M2_Wind6dof_Mir_M2S6(6) [39]/1 -> inputs/39
  MC_M2_Wind6dof_Mir_M2S5(6) [38]/1 -> inputs/38
  MC_M2_Wind6dof_Mir_M2S4(6) [37]/1 -> inputs/37
  MC_M2_Wind6dof_Mir_M2S3(6) [36]/1 -> inputs/36
  MC_M2_Wind6dof_Mir_M2S2(6) [35]/1 -> inputs/35
  MC_M2_Wind6dof_Mir_M2S1(6) [34]/1 -> inputs/34
  MC_M2_Wind6dof_Mir_M2S7(6) [33]/1 -> inputs/33
  MC_M2_Wind6dof_MacroCell(6) [32]/1 -> inputs/32
  MC_M2_Wind6dof_Cell_M2S7(6) [31]/1 -> inputs/31
  MC_M2_Wind6dof_Cell_M2S6(6) [30]/1 -> inputs/30
  MC_M2_Wind6dof_Cell_M2S5(6) [29]/1 -> inputs/29
  MC_M2_Wind6dof_Cell_M2S4(6) [28]/1 -> inputs/28
  MC_M2_Wind6dof_Cell_M2S3(6) [27]/1 -> inputs/27
  MC_M2_Wind6dof_Cell_M2S2(6) [26]/1 -> inputs/26
  MC_M2_Wind6dof_Cell_M2S1(6) [25]/1 -> inputs/25
  MC_M2_Grav_CS0(3) [24]/1 -> inputs/24
  OSS_BASE(6) [23]/1 -> inputs/23
  OSS_M2_Hex_F(6) [22]/1 -> inputs/22
  OSS_CRING_F(6) [21]/1 -> inputs/21
  OSS_TopEnd_F(6) [20]/1 -> inputs/20
  OSS_AzDrive_bot(4) [19]/1 -> inputs/19
  OSS_ElDrive_top(4) [18]/1 -> inputs/18
  OSS_ElDrive_bot(4) [17]/1 -> inputs/17
  OSS_AzDrive_top(4) [16]/1 -> inputs/16
  OSS_M1S6_cell_F(6) [15]/1 -> inputs/15
  OSS_M1S5_cell_F(6) [14]/1 -> inputs/14
  OSS_M1S4_cell_F(6) [13]/1 -> inputs/13
  OSS_M1S3_cell_F(6) [12]/1 -> inputs/12
  OSS_M1S2_cell_F(6) [11]/1 -> inputs/11
  OSS_M1S1_cell_F(6) [10]/1 -> inputs/10
  OSS_M1S7_cell_F(6) [9]/1 -> inputs/9
  OSS_M1S6_face_F(6) [8]/1 -> inputs/8
  OSS_M1S5_face_F(6) [7]/1 -> inputs/7
  OSS_M1S4_face_F(6) [6]/1 -> inputs/6
  OSS_M1S3_face_F(6) [5]/1 -> inputs/5
  OSS_M1S2_face_F(6) [4]/1 -> inputs/4
  OSS_M1S1_face_F(6) [3]/1 -> inputs/3
  OSS_M1S7_face_F(6) [2]/1 -> inputs/2
  OSS_Grav_CS0(3) [1]/1 -> inputs/1

== system AcO_Ctrl_Geometric_headless_R2016a/Structural Dynamics V3.3/Structural Dynamics V3.3/Loads ==
  " Gravity" : Constant  Value=[0;0;0]
  Base F : Constant  Value=zeros(6,1)
  Mux : Mux  Inputs=[3 102 6]
  Wind : Constant  Value=zeros(17*6,1)
  Out1 : Outport
  wires:
  Mux/1 -> Out1/1
  Base F/1 -> Mux/3
  " Gravity"/1 -> Mux/1
  Wind/1 -> Mux/2
